simulink model "sim_discrete"  (R2018a)
settings: Solver=FixedStepAuto  StartTime=0.0  StopTime=1  FixedStep=Ti  RelTol=1e-3
undefined symbols (not defined in the file): Ad, Bd, circuit, class, Co, current_correction_start, DFd, disturbance_Ro_enable, disturbance_Ro_time, disturbance_Vin_enable, disturbance_Vin_time, h, L, Ld, NFd, opt_constant_reference, opt_dead_time, opt_equilibrium_controller, opt_pwm, opt_pwm_current_controller, opt_theorem, opt_update_equilibrium, P, pwm_limit_lower, pwm_limit_upper, pwm_period, pwm_pid_kd, pwm_pid_ki, pwm_pid_kp, pwm_pid_vc_ci, pwm_pid_vc_cp, pwm_pid_vc_vi, pwm_pid_vc_vp, pwm_sample_time, Q, R, Rc, reference_controller_initial, reference_pid_ki, reference_pid_kp, Ro, Ro_p, sensor_sample, sys, Ti, Ts, Vref, Vs, Vs_p, xe
libraries: powerlib x19, simulink x19, pePwmGenerator x2
settings Model: SimulationMode=accelerator  Creator=TARCIO-FEM  LastModifiedBy=Julio-LEPO
settings OptimizationCC: EfficientMapNaN2IntZero=off
settings HardwareCC: TargetBitPerPointer=64  TargetBitPerSizeT=64  TargetBitPerPtrDiffT=64  TargetLongLongMode=on  TargetIntDivRoundTo=Zero  TargetEndianess=LittleEndian  TargetWordSize=64  TargetHWDeviceType=MATLAB Host  ProdEqTarget=off
settings CodeAppCC: MaxIdLength=128
settings GRTTargetCC: TargetLangStandard=C89/C90 (ANSI)  CombineOutputUpdateFcns=off  GRTInterface=on

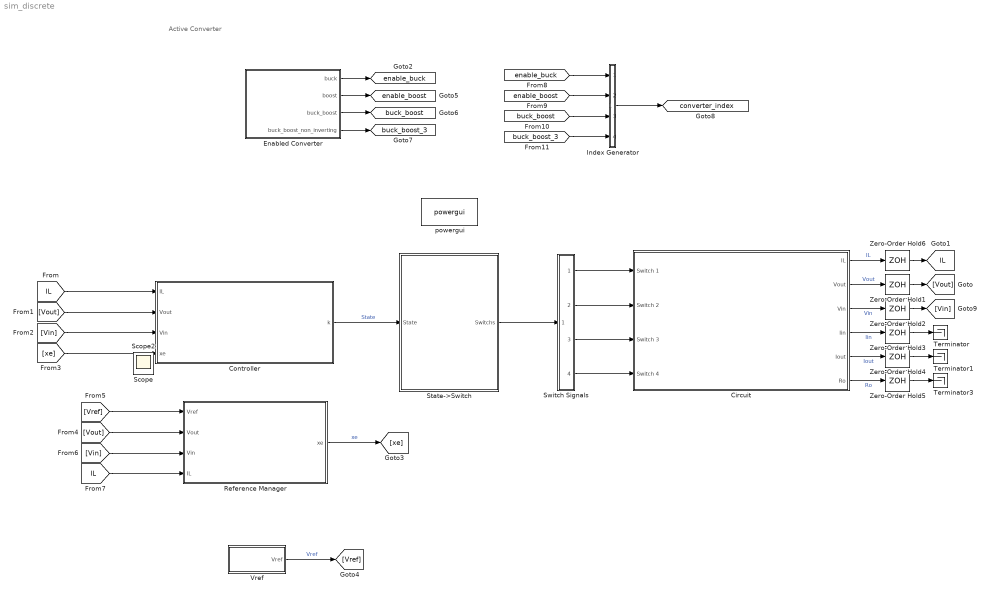
== system sim_discrete ==
  note: Active Converter
  Circuit : Subsystem
  Controller : Subsystem
  Enabled Converter : Subsystem
  Index Generator : Subsystem
  Reference Manager : Subsystem
  State->Switch : Subsystem
  Switch Signals : Subsystem
  Terminator : Terminator
  Terminator1 : Terminator
  Terminator3 : Terminator
  Vref : Subsystem
  Zero-Order Hold{1..6} (6 alike) : ZeroOrderHold  SampleTime=sensor_sample
  powergui : powerlib/powergui  Priority=1  SimulationMode=Discrete  SampleTime=Ti  frequency=60  Iterations=50  frequencyindice=0  Pbase=100e6  ErrMax=1e-4  UnitsV=kV  UnitsW=MW  buscounter=0  FunctionMessages=off  echomessages=off  EnableUseOfTLC=off  CurrentSourceSwitches=off  DisableSnubberDevices=off  DisableRonSwitches=off  DisableVfSwitches=off  DisplayEquations=off  SolverType=Tustin/Backward Euler (TBE)  Interpol=off  ExternalGateDelay=off  methode=off  Ts=100  x0status=blocks  SPID=off  SwTol=0  HookPort=off  RestoreLinks=warning  ResistiveCurrentMeasurement=off  Frange=[0:2:500]  Ylog=off  Xlog=on  ShowGrid=off  save=off  variable=ZData  structure=0  ZoomFFT=off  StartTime=0.0  cycles=1  DisplayStyle=1  fundamental=60  FreqAxis=off  MaxFrequency=1000  frequencyindicesteady=1  RmsSteady=1  display=off
  Scope : Scope
  Scope2 : Scope
  tag scope: IL=global, buck_boost=global, buck_boost_3=global, converter_index=global, enable_boost=global, enable_buck=global
  wires:
  Controller/1(k) -> State->Switch/1(State)  "State"
  [IL] -> Controller/1(IL)
  [xe] -> Controller/4(xe)
  [Vin] -> Controller/3(Vin)
  [Vout] -> Controller/2(Vout)
  Reference Manager/1(xe) -> [xe]  "xe"
  Index Generator/1(Out1) -> [converter_index]
  [Vout] -> Reference Manager/2(Vout)
  Circuit/5(Iout) -> Zero-Order Hold4/1  "Iout"
  Zero-Order Hold2/1 -> [Vin]
  Enabled Converter/3(buck_boost) -> [buck_boost]
  Switch Signals/3(S3) -> Circuit/3(Switch 3)
  [buck_boost_3] -> Index Generator/4(In4)
  Circuit/3(Vin) -> Zero-Order Hold2/1  "Vin"
  Circuit/1(IL) -> Zero-Order Hold6/1  "IL"
  Switch Signals/2(S2) -> Circuit/2(Switch 2)
  Circuit/6(Ro) -> Zero-Order Hold5/1  "Ro"
  Enabled Converter/2(boost) -> [enable_boost]
  [IL] -> Reference Manager/4(IL)
  [enable_buck] -> Index Generator/1(In1)
  [Vref] -> Reference Manager/1(Vref)
  Circuit/2(Vout) -> Zero-Order Hold1/1  "Vout"
  State->Switch/1(Switchs) -> Switch Signals/1(In1)
  Zero-Order Hold5/1 -> Terminator3/1
  Zero-Order Hold3/1 -> Terminator/1
  Switch Signals/4(S4) -> Circuit/4(Switch 4)
  Zero-Order Hold1/1 -> [Vout]
  Switch Signals/1(S1) -> Circuit/1(Switch 1)
  Vref/1(Vref) -> [Vref]  "Vref"
  Zero-Order Hold6/1 -> [IL]
  Circuit/4(Iin) -> Zero-Order Hold3/1  "Iin"
  Zero-Order Hold4/1 -> Terminator1/1
  Enabled Converter/4(buck_boost_non_inverting) -> [buck_boost_3]
  Enabled Converter/1(buck) -> [enable_buck]
  [Vin] -> Reference Manager/3(Vin)
  [enable_boost] -> Index Generator/2(In2)
  [buck_boost] -> Index Generator/3(In3)

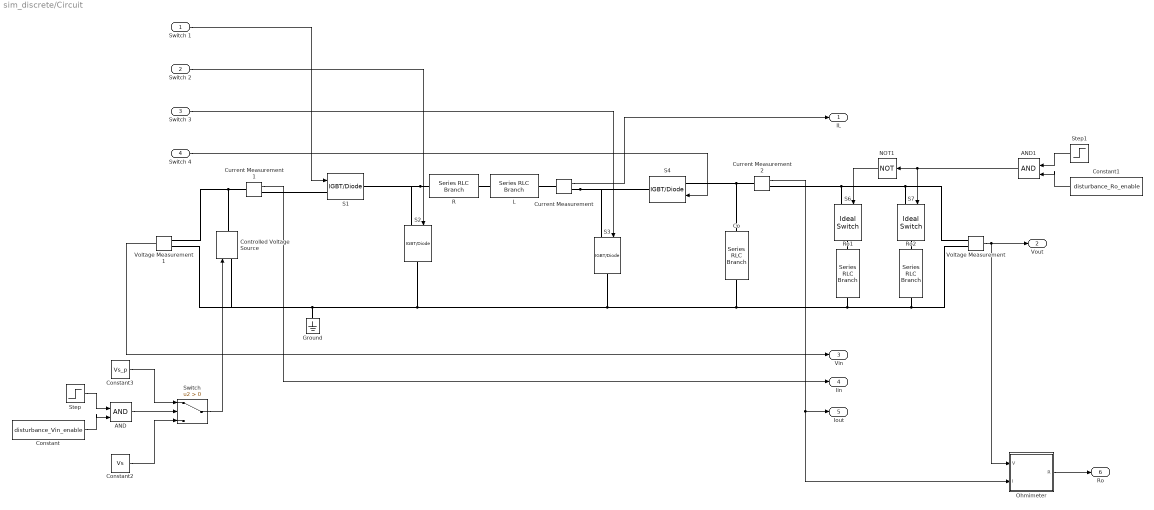
== system sim_discrete/Circuit ==
  Switch 1 : Inport
  Switch 2 : Inport  Port=2
  Switch 3 : Inport  Port=3
  Switch 4 : Inport  Port=4
  AND : Logic  IconShape=distinctive  AllPortsSameDT=off  OutDataTypeStr=boolean
  AND1 : Logic  IconShape=distinctive  AllPortsSameDT=off  OutDataTypeStr=boolean
  Co : powerlib/Elements/Series RLC Branch  LConnTagsString=__new0  RConnTagsString=__new0  BranchType=RC  Resistance=Rc  Inductance=L  SetiL0=off  InitialCurrent=0  Capacitance=Co  Setx0=off  InitialVoltage=0  Measurements=None
  Constant : Constant  Value=disturbance_Vin_enable
  Constant1 : Constant  Value=disturbance_Ro_enable
  Constant2 : Constant  Value=Vs
  Constant3 : Constant  Value=Vs_p
  Controlled Voltage Source : powerlib/Electrical Sources/Controlled Voltage Source  Initialize=on  Source_Type=DC  Amplitude=0  Phase=0  Frequency=0  Measurements=None
  Current Measurement : powerlib/Measurements/Current Measurement  PhasorSimulation=off  OutputType=Complex  PSBequivalent=0
  Current Measurement1 : powerlib/Measurements/Current Measurement  PhasorSimulation=off  OutputType=Complex  PSBequivalent=0
  Current Measurement2 : powerlib/Measurements/Current Measurement  PhasorSimulation=off  OutputType=Complex  PSBequivalent=0
  Ground : powerlib/Elements/Ground  LConnTagsString=a
  L : powerlib/Elements/Series RLC Branch  LConnTagsString=__new0  RConnTagsString=__new0  BranchType=L  Resistance=1  Inductance=L  SetiL0=off  InitialCurrent=0  Capacitance=1e-6  Setx0=off  InitialVoltage=0  Measurements=None
  NOT1 : Logic  Operator=NOT  IconShape=distinctive  AllPortsSameDT=off  OutDataTypeStr=boolean
  Ohmimeter : Subsystem
  R : powerlib/Elements/Series RLC Branch  LConnTagsString=__new0  RConnTagsString=__new0  BranchType=R  Resistance=R  Inductance=1e-3  SetiL0=off  InitialCurrent=0  Capacitance=1e-6  Setx0=off  InitialVoltage=0  Measurements=None
  Ro1 : powerlib/Elements/Series RLC Branch  LConnTagsString=__new0  RConnTagsString=__new0  BranchType=R  Resistance=Ro  Inductance=1e-3  SetiL0=off  InitialCurrent=0  Capacitance=1e-6  Setx0=off  InitialVoltage=0  Measurements=None
  Ro2 : powerlib/Elements/Series RLC Branch  LConnTagsString=__new0  RConnTagsString=__new0  BranchType=R  Resistance=Ro_p  Inductance=1e-3  SetiL0=off  InitialCurrent=0  Capacitance=1e-6  Setx0=off  InitialVoltage=0  Measurements=None
  S{1..4} (4 alike) : powerlib/Power Electronics/IGBT//Diode  Ron=1e-3  Rs=1e5  Cs=inf  Measurements=off
  S6 : powerlib/Power Electronics/Ideal Switch  Ron=0.001  Lon=0  IC=0  Rs=1e5  Cs=inf  Measurements=off
  S7 : powerlib/Power Electronics/Ideal Switch  Ron=0.001  Lon=0  IC=0  Rs=1e5  Cs=inf  Measurements=off
  Step : Step  Time=disturbance_Vin_time  SampleTime=0
  Step1 : Step  Time=disturbance_Ro_time  SampleTime=0
  Switch : Switch  Criteria=u2 > Threshold
  Voltage Measurement : powerlib/Measurements/Voltage Measurement  PhasorSimulation=off  OutputType=Complex  PSBequivalent=0
  Voltage Measurement1 : powerlib/Measurements/Voltage Measurement  PhasorSimulation=off  OutputType=Complex  PSBequivalent=0
  IL : Outport
  Vout : Outport  Port=2
  Vin : Outport  Port=3
  Iin : Outport  Port=4
  Iout : Outport  Port=5
  Ro : Outport  Port=6
  wires:
  Switch 1/1 -> S1/1
  Voltage Measurement1/1 -> Vin/1
  Switch 2/1 -> S2/1
  Constant1/1 -> AND1/2
  AND1/1 -> S7/1, NOT1/1
  NOT1/1 -> S6/1
  Step1/1 -> AND1/1
  AND/1 -> Switch/2
  Constant/1 -> AND/2
  Step/1 -> AND/1
  Constant2/1 -> Switch/3
  Constant3/1 -> Switch/1
  Current Measurement1/1 -> Iin/1
  Current Measurement/1 -> IL/1
  Switch/1 -> Controlled Voltage Source/1
  Switch 4/1 -> S4/1
  Switch 3/1 -> S3/1
  Voltage Measurement/1 -> Vout/1, Ohmimeter/1(V)
  Ohmimeter/1(R) -> Ro/1
  Current Measurement2/1 -> Ohmimeter/2(I), Iout/1
  connections:
  L/LConn1 -- R/RConn1
  R/LConn1 -- S2/LConn1 -- S1/RConn1
  Current Measurement/LConn1 -- L/RConn1
  Current Measurement2/LConn1 -- S4/LConn1 -- Co/LConn1
  Voltage Measurement/LConn2 -- Ro2/RConn1 -- Ro1/RConn1 -- S3/RConn1 -- S2/RConn1 -- Voltage Measurement1/LConn2 -- Controlled Voltage Source/LConn1 -- Ground/LConn1 -- Co/RConn1
  S7/RConn1 -- Ro2/LConn1
  S6/RConn1 -- Ro1/LConn1
  Current Measurement1/LConn1 -- Controlled Voltage Source/RConn1 -- Voltage Measurement1/LConn1
  S1/LConn1 -- Current Measurement1/RConn1
  S6/LConn1 -- Current Measurement2/RConn1 -- S7/LConn1 -- Voltage Measurement/LConn1
  Current Measurement/RConn1 -- S4/RConn1 -- S3/LConn1

== system sim_discrete/Controller ==
  IL : Inport
  Vout : Inport  Port=2
  Vin : Inport  Port=3
  xe : Inport  Port=4
  Constant : Constant  Value=opt_pwm
  Discrete Switched Control : Subsystem
  PWM Control : Subsystem
  Selector : Selector  InputPortWidth=2  IndexOptions=Index vector (dialog)  Indices=[2]  OutputSizes=1
  Switch : Switch  Criteria=u2 > Threshold
  k : Outport
  wires:
  IL/1 -> PWM Control/3(IL), Discrete Switched Control/1(IL)
  Vout/1 -> PWM Control/2(Vout), Discrete Switched Control/2(Vout)
  Vin/1 -> Discrete Switched Control/3(Vin)
  Switch/1 -> k/1
  Discrete Switched Control/1(k) -> Switch/3  "Switched Control K"
  Constant/1 -> Switch/2
  xe/1 -> Discrete Switched Control/4(xe), Selector/1
  Selector/1 -> PWM Control/1(Vref)
  PWM Control/1(k) -> Switch/1  "PWM K"

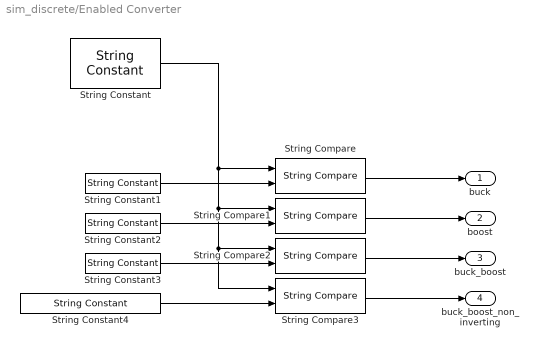
== system sim_discrete/Enabled Converter ==
  String Compare{,1..3} (4 alike) : StringCompare
  String Constant : StringConstant  String=class(circuit)
  String Constant1 : StringConstant  String='buck'
  String Constant2 : StringConstant  String='boost'
  String Constant3 : StringConstant  String='buck_boost'
  String Constant4 : StringConstant  String='buck_boost_non_inverting'
  buck : Outport
  boost : Outport  Port=2
  buck_boost : Outport  Port=3
  buck_boost_non_inverting : Outport  Port=4
  wires:
  String Constant1/1 -> String Compare/2
  String Constant/1 -> String Compare/1, String Compare1/1, String Compare2/1, String Compare3/1
  String Constant3/1 -> String Compare2/2
  String Compare2/1 -> buck_boost/1
  String Compare1/1 -> boost/1
  String Constant4/1 -> String Compare3/2
  String Compare3/1 -> buck_boost_non_inverting/1
  String Compare/1 -> buck/1
  String Constant2/1 -> String Compare1/2

== system sim_discrete/Index Generator ==
  In1 : Inport
  In2 : Inport  Port=2
  In3 : Inport  Port=3
  In4 : Inport  Port=4
  Gain : Gain
  Gain1 : Gain  Gain=2
  Gain2 : Gain  Gain=3
  Gain3 : Gain  Gain=4
  Sum : Sum  Inputs=++++
  Out1 : Outport
  wires:
  Gain/1 -> Sum/1
  In3/1 -> Gain2/1
  In2/1 -> Gain1/1
  Gain1/1 -> Sum/2
  Sum/1 -> Out1/1
  Gain2/1 -> Sum/3
  In4/1 -> Gain3/1
  Gain3/1 -> Sum/4
  In1/1 -> Gain/1

== system sim_discrete/Reference Manager ==
  Vref : Inport
  Vout : Inport  Port=2
  Vin : Inport  Port=3
  IL : Inport  Port=4
  Constant : Constant  Value=xe
  Reference Update : Subsystem
  Switch : Switch  Criteria=u2 > Threshold
  opt_update_equilibrium : Constant  Value=opt_update_equilibrium
  xe : Outport
  wires:
  Vout/1 -> Reference Update/2(Vout)
  Vin/1 -> Reference Update/3(Vin)
  Vref/1 -> Reference Update/1(Vref)
  opt_update_equilibrium/1 -> Switch/2
  Switch/1 -> xe/1
  Reference Update/1(xe) -> Switch/1  "xe"
  Constant/1 -> Switch/3
  IL/1 -> Reference Update/4(IL)

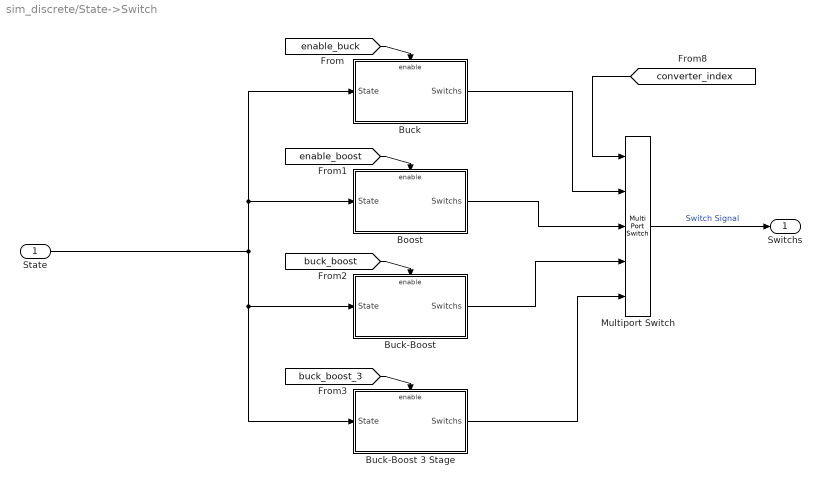
== system sim_discrete/State->Switch ==
  State : Inport
  Boost : Subsystem
  Buck : Subsystem
  Buck-Boost : Subsystem
  Buck-Boost 3 Stage : Subsystem
  Multiport Switch : MultiPortSwitch  Inputs=4
  Switchs : Outport
  wires:
  State/1 -> Buck-Boost/1(State), Buck-Boost 3 Stage/1(State), Boost/1(State), Buck/1(State)
  Buck/1(Switchs) -> Multiport Switch/2
  Boost/1(Switchs) -> Multiport Switch/3
  Buck-Boost 3 Stage/1(Switchs) -> Multiport Switch/5
  Buck-Boost/1(Switchs) -> Multiport Switch/4
  [enable_buck] -> Buck/Enable
  [enable_boost] -> Boost/Enable
  [buck_boost] -> Buck-Boost/Enable
  [buck_boost_3] -> Buck-Boost 3 Stage/Enable
  Multiport Switch/1 -> Switchs/1  "Switch Signal"
  [converter_index] -> Multiport Switch/1

== system sim_discrete/Switch Signals ==
  In1 : Inport
  Constant : Constant  Value=opt_dead_time
  Dead Time : Subsystem
  Demux : Demux
  Scope : Scope  NumInputPorts=2
  Switch : Switch  Criteria=u2 > Threshold
  S1 : Outport
  S2 : Outport  Port=2
  S3 : Outport  Port=3
  S4 : Outport  Port=4
  wires:
  Constant/1 -> Dead Time/Enable, Switch/2
  Dead Time/1(Out1) -> Scope/2, Switch/1
  In1/1 -> Scope/1, Dead Time/1(In1), Switch/3
  Demux/2 -> S2/1
  Demux/1 -> S1/1
  Demux/4 -> S4/1
  Demux/3 -> S3/1
  Switch/1 -> Demux/1

== system sim_discrete/Vref ==
  Constant Reference : Subsystem
  Switch1 : Switch  Criteria=u2 > Threshold
  Variable Reference : Subsystem
  opt_constant_reference : Constant  Value=opt_constant_reference
  Vref : Outport
  wires:
  opt_constant_reference/1 -> Switch1/2
  Switch1/1 -> Vref/1
  Variable Reference/1(Vref) -> Switch1/3
  Constant Reference/1(Vref) -> Switch1/1

== system sim_discrete/Circuit/Ohmimeter ==
  V : Inport
  I : Inport  Port=2
  Compare To Zero : simulink/Logic and Bit Operations/Compare To Zero  relop=~=  OutDataTypeStr=boolean
  Constant4 : Constant  Value=Ro
  Divide : Product  Inputs=*/
  One : Constant
  Switch1 : Switch  Criteria=u2 ~= 0
  Switch2 : Switch  Criteria=u2 ~= 0
  R : Outport
  wires:
  Compare To Zero/1 -> Switch1/2, Switch2/2
  I/1 -> Switch1/1, Compare To Zero/1
  Divide/1 -> Switch2/1
  Constant4/1 -> Switch2/3
  Switch1/1 -> Divide/2
  One/1 -> Switch1/3
  V/1 -> Divide/1
  Switch2/1 -> R/1

== system sim_discrete/Controller/Discrete Switched Control ==
  IL : Inport
  Vout : Inport  Port=2
  Vin : Inport  Port=3
  xe : Inport  Port=4
  Discrete Switching Strategy : MATLAB Function  TreatAsAtomicUnit=on
  Mux : Mux  Inputs=2
  System Properties : Subsystem
  Zero-Order Hold : ZeroOrderHold  SampleTime=Ts
  k : Outport
  wires:
  Vin/1 -> Discrete Switching Strategy/4(u)
  Discrete Switching Strategy/1(k) -> Zero-Order Hold/1
  System Properties/1(theorem) -> Discrete Switching Strategy/1(theorem)
  System Properties/2(sys) -> Discrete Switching Strategy/2(sys)
  Mux/1 -> Discrete Switching Strategy/3(x)
  IL/1 -> Mux/1
  Vout/1 -> Mux/2
  xe/1 -> Discrete Switching Strategy/5(xe)
  Zero-Order Hold/1 -> k/1

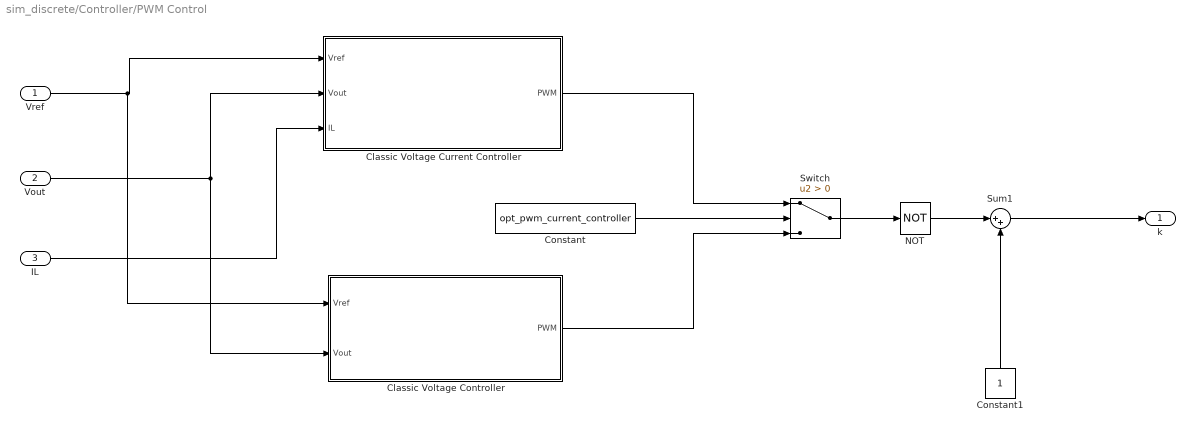
== system sim_discrete/Controller/PWM Control ==
  Vref : Inport
  Vout : Inport  Port=2
  IL : Inport  Port=3
  Classic Voltage Controller : Subsystem
  Classic Voltage Current Controller : Subsystem
  Constant : Constant  Value=opt_pwm_current_controller
  Constant1 : Constant
  NOT : Logic  Operator=NOT  IconShape=distinctive  AllPortsSameDT=off  OutDataTypeStr=boolean
  Sum1 : Sum  Inputs=|++
  Switch : Switch  Criteria=u2 > Threshold
  k : Outport
  wires:
  Sum1/1 -> k/1
  NOT/1 -> Sum1/1
  Constant1/1 -> Sum1/2
  Vref/1 -> Classic Voltage Controller/1(Vref), Classic Voltage Current Controller/1(Vref)
  Vout/1 -> Classic Voltage Controller/2(Vout), Classic Voltage Current Controller/2(Vout)
  IL/1 -> Classic Voltage Current Controller/3(IL)
  Constant/1 -> Switch/2
  Switch/1 -> NOT/1
  Classic Voltage Controller/1(PWM) -> Switch/3
  Classic Voltage Current Controller/1(PWM) -> Switch/1

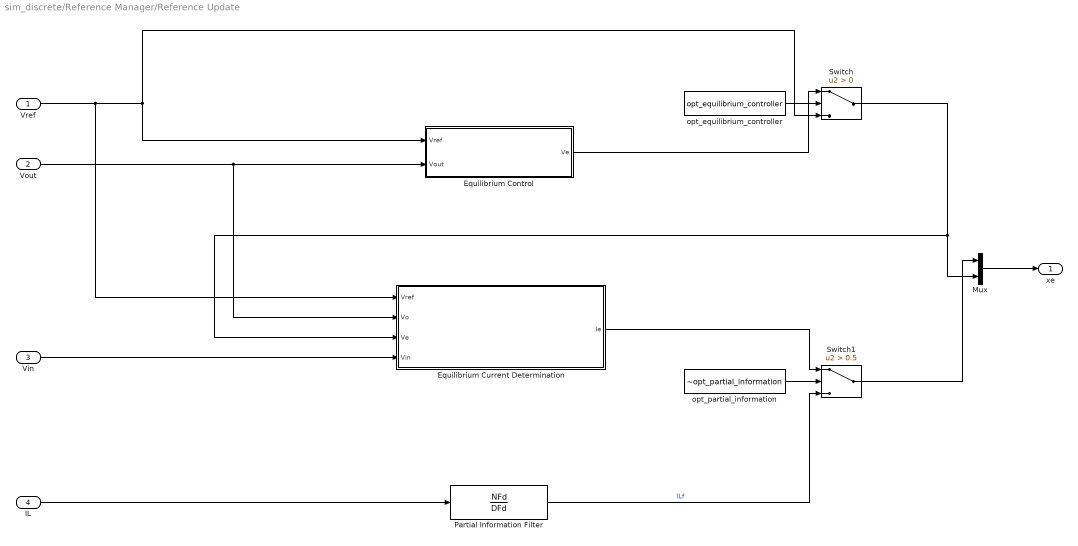
== system sim_discrete/Reference Manager/Reference Update ==
  Vref : Inport
  Vout : Inport  Port=2
  Vin : Inport  Port=3
  IL : Inport  Port=4
  Equilibrium Control : Subsystem
  Equilibrium Current Determination : Subsystem
  Mux : Mux  Inputs=2
  Partial Information Filter : DiscreteTransferFcn  Numerator=NFd  Denominator=DFd  SampleTime=1e-3
  Switch : Switch  Criteria=u2 > Threshold
  Switch1 : Switch  Criteria=u2 > Threshold  Threshold=0.5
  opt_equilibrium_controller : Constant  Value=opt_equilibrium_controller
  opt_partial_information : Constant  Value=~opt_partial_information
  xe : Outport
  wires:
  Vref/1 -> Equilibrium Current Determination/1(Vref), Equilibrium Control/1(Vref), Switch/3
  Mux/1 -> xe/1
  opt_equilibrium_controller/1 -> Switch/2
  Switch/1 -> Equilibrium Current Determination/3(Ve), Mux/2
  Switch1/1 -> Mux/1
  opt_partial_information/1 -> Switch1/2
  Partial Information Filter/1 -> Switch1/3  "ILf"
  IL/1 -> Partial Information Filter/1
  Vout/1 -> Equilibrium Current Determination/2(Vo), Equilibrium Control/2(Vout)
  Equilibrium Control/1(Ve) -> Switch/1
  Vin/1 -> Equilibrium Current Determination/4(Vin)
  Equilibrium Current Determination/1(Ie) -> Switch1/1

== system sim_discrete/State->Switch/Boost ==
  State : Inport
  Enable : EnablePort
  Compare To Constant : simulink/Logic and Bit Operations/Compare To Constant  relop=<=  const=1.5  OutDataTypeStr=boolean
  Constant : Constant  Value=false
  Constant1 : Constant  Value=true
  Mux : Mux
  NOT : Logic  Operator=NOT  IconShape=distinctive  AllPortsSameDT=off  OutDataTypeStr=boolean
  Switchs : Outport
  wires:
  Mux/1 -> Switchs/1
  Compare To Constant/1 -> Mux/3, NOT/1
  State/1 -> Compare To Constant/1
  NOT/1 -> Mux/4
  Constant1/1 -> Mux/1
  Constant/1 -> Mux/2

== system sim_discrete/State->Switch/Buck ==
  State : Inport
  Enable : EnablePort
  Compare To Constant : simulink/Logic and Bit Operations/Compare To Constant  relop=<=  const=1.5  OutDataTypeStr=boolean
  Constant : Constant  Value=false
  Constant1 : Constant  Value=true
  Mux : Mux
  NOT : Logic  Operator=NOT  IconShape=distinctive  AllPortsSameDT=off  OutDataTypeStr=boolean
  Switchs : Outport
  wires:
  Mux/1 -> Switchs/1
  Compare To Constant/1 -> Mux/1, NOT/1
  Constant1/1 -> Mux/4
  NOT/1 -> Mux/2
  Constant/1 -> Mux/3
  State/1 -> Compare To Constant/1

== system sim_discrete/State->Switch/Buck-Boost ==
  State : Inport
  Enable : EnablePort
  Compare To Constant : simulink/Logic and Bit Operations/Compare To Constant  relop=<=  const=1.5  OutDataTypeStr=boolean
  Mux : Mux
  NOT : Logic  Operator=NOT  IconShape=distinctive  AllPortsSameDT=off  OutDataTypeStr=boolean
  Switchs : Outport
  wires:
  Mux/1 -> Switchs/1
  Compare To Constant/1 -> Mux/3, Mux/1, NOT/1
  NOT/1 -> Mux/4, Mux/2
  State/1 -> Compare To Constant/1

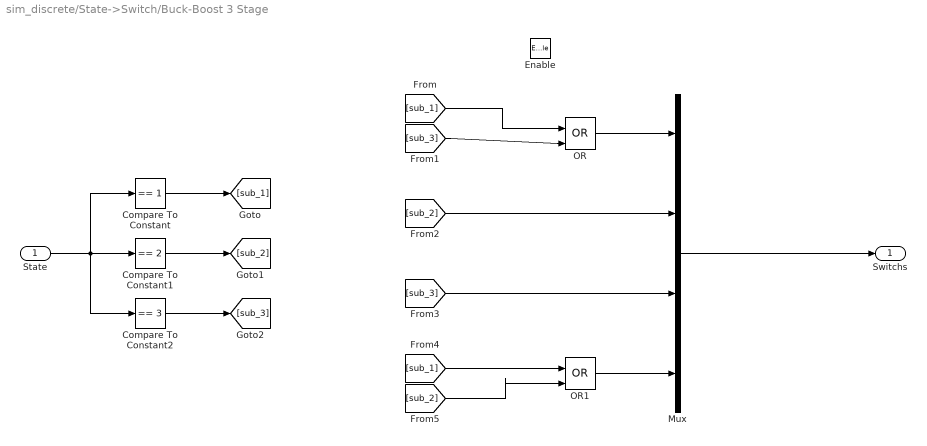
== system sim_discrete/State->Switch/Buck-Boost 3 Stage ==
  State : Inport
  Enable : EnablePort
  Compare To Constant : simulink/Logic and Bit Operations/Compare To Constant  relop===  const=1  OutDataTypeStr=boolean
  Compare To Constant1 : simulink/Logic and Bit Operations/Compare To Constant  relop===  const=2  OutDataTypeStr=boolean
  Compare To Constant2 : simulink/Logic and Bit Operations/Compare To Constant  relop===  const=3  OutDataTypeStr=boolean
  Mux : Mux
  OR : Logic  Operator=OR  IconShape=distinctive  AllPortsSameDT=off  OutDataTypeStr=boolean
  OR1 : Logic  Operator=OR  IconShape=distinctive  AllPortsSameDT=off  OutDataTypeStr=boolean
  Switchs : Outport
  wires:
  Mux/1 -> Switchs/1
  [sub_1] -> OR/1
  [sub_1] -> OR1/1
  [sub_2] -> Mux/2
  [sub_2] -> OR1/2
  State/1 -> Compare To Constant2/1, Compare To Constant1/1, Compare To Constant/1
  OR1/1 -> Mux/4
  [sub_3] -> OR/2
  [sub_3] -> Mux/3
  Compare To Constant/1 -> [sub_1]
  Compare To Constant2/1 -> [sub_3]
  OR/1 -> Mux/1
  Compare To Constant1/1 -> [sub_2]

== system sim_discrete/Switch Signals/Dead Time ==
  In1 : Inport
  Enable : EnablePort
  Dead Time : Subsystem
  Dead Time1 : Subsystem
  Dead Time2 : Subsystem
  Dead Time3 : Subsystem
  Demux : Demux
  Mux : Mux
  Out1 : Outport
  wires:
  Demux/4 -> Dead Time3/1(Signal)
  Demux/3 -> Dead Time2/1(Signal)
  Demux/2 -> Dead Time1/1(Signal)
  Demux/1 -> Dead Time/1(Signal)
  In1/1 -> Demux/1
  Dead Time3/1(Signal Delayed) -> Mux/4
  Dead Time2/1(Signal Delayed) -> Mux/3
  Dead Time1/1(Signal Delayed) -> Mux/2
  Dead Time/1(Signal Delayed) -> Mux/1
  Mux/1 -> Out1/1

== system sim_discrete/Vref/Constant Reference ==
  Constant : Constant  Value=Vref
  Vref : Outport
  wires:
  Constant/1 -> Vref/1

== system sim_discrete/Vref/Variable Reference ==
  Constant : Constant  Value=Vref
  Rate Limiter : RateLimiter  RisingSlewLimit=10  FallingSlewLimit=-10  SampleTimeMode=inherited
  Step : Step  Time=1.5  After=20  SampleTime=0
  Sum : Sum  Inputs=|++
  Vref : Outport
  wires:
  Constant/1 -> Sum/1
  Sum/1 -> Vref/1
  Step/1 -> Rate Limiter/1
  Rate Limiter/1 -> Sum/2

== system sim_discrete/Controller/Discrete Switched Control/System Properties ==
  Bus Creator : BusCreator  Inputs=7  OutDataTypeStr=Bus: SystemDataBus
  Constant : Constant  Value=Ad  VectorParams1D=off
  Constant1 : Constant  Value=Bd  VectorParams1D=off
  Constant2 : Constant  Value=P  VectorParams1D=off
  Constant3 : Constant  Value=Q  VectorParams1D=off
  Constant4 : Constant  Value=h  VectorParams1D=off
  Constant5 : Constant  Value=sys.N
  Constant6 : Constant  Value=opt_theorem
  Constant7 : Constant  Value=Ld  VectorParams1D=off
  theorem : Outport
  sys : Outport  Port=2
  wires:
  Bus Creator/1 -> sys/1
  Constant2/1 -> Bus Creator/3  "P"
  Constant1/1 -> Bus Creator/2  "B"
  Constant/1 -> Bus Creator/1  "A"
  Constant3/1 -> Bus Creator/4  "Q"
  Constant5/1 -> Bus Creator/5  "N"
  Constant6/1 -> theorem/1
  Constant4/1 -> Bus Creator/6  "h"
  Constant7/1 -> Bus Creator/7  "L"

== system sim_discrete/Controller/PWM Control/Classic Voltage Controller ==
  Vref : Inport
  Vout : Inport  Port=2
  PID Controller : simulink/Continuous/PID Controller  Controller=PI  TimeDomain=Discrete-time  SampleTime=pwm_period  IntegratorMethod=Forward Euler  FilterMethod=Forward Euler  Form=Parallel  UseFilter=on  ControllerParametersSource=internal  P=pwm_pid_kp  I=pwm_pid_ki  D=pwm_pid_kd  N=100  InitialConditionSource=internal  InitialConditionForIntegrator=0  InitialConditionForFilter=0  ExternalReset=none  LimitOutput=off  UpperSaturationLimit=inf  LowerSaturationLimit=-inf  LinearizeAsGain=on  AntiWindupMode=none  Kb=1  TrackingMode=off  Kt=1  PParamMin=[]  PParamMax=[]  IParamMin=[]  IParamMax=[]  DParamMin=[]  DParamMax=[]  NParamMin=[]  NParamMax=[]  KbParamMin=[]  KbParamMax=[]  KtParamMin=[]  KtParamMax=[]  POutMin=[]  POutMax=[]  IOutMin=[]  IOutMax=[]  DOutMin=[]  DOutMax=[]  NOutMin=[]  NOutMax=[]  KbOutMin=[]  KbOutMax=[]  KtOutMin=[]  KtOutMax=[]  IntegratorOutMin=[]  IntegratorOutMax=[]  FilterOutMin=[]  FilterOutMax=[]  SumOutMin=[]  SumOutMax=[]  SumI1OutMin=[]  SumI1OutMax=[]  SumI2OutMin=[]  SumI2OutMax=[]  SumI3OutMin=[]  SumI3OutMax=[]  SumDOutMin=[]  SumDOutMax=[]  SaturationOutMin=[]  SaturationOutMax=[]  IntegratorContinuousStateAttributes=''  IntegratorStateMustResolveToSignalObject=off  IntegratorRTWStateStorageClass=Auto  FilterContinuousStateAttributes=''  FilterStateMustResolveToSignalObject=off  FilterRTWStateStorageClass=Auto  DifferentiatorICPrevScaledInput=0  DifferentiatorOutMin=[]  DifferentiatorOutMax=[]  FilterDiffOutCoefMin=[]  FilterDiffOutCoefMax=[]  SumDenOutMin=[]  SumDenOutMax=[]  SumNumOutMin=[]  SumNumOutMax=[]  ReciprocalOutMin=[]  ReciprocalOutMax=[]  DivideOutMin=[]  DivideOutMax=[]  TunerSelectOption=Transfer Function Based (PID Tuner App)
  PWM Generator : pePwmGenerator/PWM Generator  CarrCount=Up  Tper=pwm_period  Ts=pwm_sample_time
  Saturation : Saturate  UpperLimit=pwm_limit_upper  LowerLimit=pwm_limit_lower
  Sum : Sum  Inputs=|+-
  PWM : Outport
  wires:
  Saturation/1 -> PWM Generator/1  "PWM Duty Cycle"
  PWM Generator/1 -> PWM/1
  PID Controller/1 -> Saturation/1
  Sum/1 -> PID Controller/1
  Vref/1 -> Sum/1
  Vout/1 -> Sum/2

== system sim_discrete/Controller/PWM Control/Classic Voltage Current Controller ==
  Vref : Inport
  Vout : Inport  Port=2
  IL : Inport  Port=3
  Current Controller : simulink/Continuous/PID Controller  Controller=PI  TimeDomain=Discrete-time  SampleTime=pwm_period  IntegratorMethod=Forward Euler  FilterMethod=Forward Euler  Form=Parallel  UseFilter=on  ControllerParametersSource=internal  P=pwm_pid_vc_cp  I=pwm_pid_vc_ci  D=pwm_pid_kd  N=100  InitialConditionSource=internal  InitialConditionForIntegrator=0  InitialConditionForFilter=0  ExternalReset=none  LimitOutput=off  UpperSaturationLimit=inf  LowerSaturationLimit=-inf  LinearizeAsGain=on  AntiWindupMode=none  Kb=1  TrackingMode=off  Kt=1  PParamMin=[]  PParamMax=[]  IParamMin=[]  IParamMax=[]  DParamMin=[]  DParamMax=[]  NParamMin=[]  NParamMax=[]  KbParamMin=[]  KbParamMax=[]  KtParamMin=[]  KtParamMax=[]  POutMin=[]  POutMax=[]  IOutMin=[]  IOutMax=[]  DOutMin=[]  DOutMax=[]  NOutMin=[]  NOutMax=[]  KbOutMin=[]  KbOutMax=[]  KtOutMin=[]  KtOutMax=[]  IntegratorOutMin=[]  IntegratorOutMax=[]  FilterOutMin=[]  FilterOutMax=[]  SumOutMin=[]  SumOutMax=[]  SumI1OutMin=[]  SumI1OutMax=[]  SumI2OutMin=[]  SumI2OutMax=[]  SumI3OutMin=[]  SumI3OutMax=[]  SumDOutMin=[]  SumDOutMax=[]  SaturationOutMin=[]  SaturationOutMax=[]  IntegratorContinuousStateAttributes=''  IntegratorStateMustResolveToSignalObject=off  IntegratorRTWStateStorageClass=Auto  FilterContinuousStateAttributes=''  FilterStateMustResolveToSignalObject=off  FilterRTWStateStorageClass=Auto  DifferentiatorICPrevScaledInput=0  DifferentiatorOutMin=[]  DifferentiatorOutMax=[]  FilterDiffOutCoefMin=[]  FilterDiffOutCoefMax=[]  SumDenOutMin=[]  SumDenOutMax=[]  SumNumOutMin=[]  SumNumOutMax=[]  ReciprocalOutMin=[]  ReciprocalOutMax=[]  DivideOutMin=[]  DivideOutMax=[]  TunerSelectOption=Transfer Function Based (PID Tuner App)
  PWM Generator : pePwmGenerator/PWM Generator  CarrCount=Up  Tper=pwm_period  Ts=pwm_sample_time
  Saturation : Saturate  UpperLimit=pwm_limit_upper  LowerLimit=pwm_limit_lower
  Sum : Sum  Inputs=|+-
  Sum2 : Sum  Inputs=|+-
  Voltage Controller : simulink/Continuous/PID Controller  Controller=PI  TimeDomain=Discrete-time  SampleTime=pwm_period  IntegratorMethod=Forward Euler  FilterMethod=Forward Euler  Form=Parallel  UseFilter=on  ControllerParametersSource=internal  P=pwm_pid_vc_vp  I=pwm_pid_vc_vi  D=0  N=100  InitialConditionSource=internal  InitialConditionForIntegrator=0  InitialConditionForFilter=0  ExternalReset=none  LimitOutput=off  UpperSaturationLimit=inf  LowerSaturationLimit=-inf  LinearizeAsGain=on  AntiWindupMode=none  Kb=1  TrackingMode=off  Kt=1  PParamMin=[]  PParamMax=[]  IParamMin=[]  IParamMax=[]  DParamMin=[]  DParamMax=[]  NParamMin=[]  NParamMax=[]  KbParamMin=[]  KbParamMax=[]  KtParamMin=[]  KtParamMax=[]  POutMin=[]  POutMax=[]  IOutMin=[]  IOutMax=[]  DOutMin=[]  DOutMax=[]  NOutMin=[]  NOutMax=[]  KbOutMin=[]  KbOutMax=[]  KtOutMin=[]  KtOutMax=[]  IntegratorOutMin=[]  IntegratorOutMax=[]  FilterOutMin=[]  FilterOutMax=[]  SumOutMin=[]  SumOutMax=[]  SumI1OutMin=[]  SumI1OutMax=[]  SumI2OutMin=[]  SumI2OutMax=[]  SumI3OutMin=[]  SumI3OutMax=[]  SumDOutMin=[]  SumDOutMax=[]  SaturationOutMin=[]  SaturationOutMax=[]  IntegratorContinuousStateAttributes=''  IntegratorStateMustResolveToSignalObject=off  IntegratorRTWStateStorageClass=Auto  FilterContinuousStateAttributes=''  FilterStateMustResolveToSignalObject=off  FilterRTWStateStorageClass=Auto  DifferentiatorICPrevScaledInput=0  DifferentiatorOutMin=[]  DifferentiatorOutMax=[]  FilterDiffOutCoefMin=[]  FilterDiffOutCoefMax=[]  SumDenOutMin=[]  SumDenOutMax=[]  SumNumOutMin=[]  SumNumOutMax=[]  ReciprocalOutMin=[]  ReciprocalOutMax=[]  DivideOutMin=[]  DivideOutMax=[]  TunerSelectOption=Transfer Function Based (PID Tuner App)
  PWM : Outport
  wires:
  Sum2/1 -> Current Controller/1
  Sum/1 -> Voltage Controller/1
  Vout/1 -> Sum/2
  Voltage Controller/1 -> Sum2/1
  IL/1 -> Sum2/2
  Current Controller/1 -> Saturation/1
  Vref/1 -> Sum/1
  Saturation/1 -> PWM Generator/1  "PWM Duty Cycle"
  PWM Generator/1 -> PWM/1

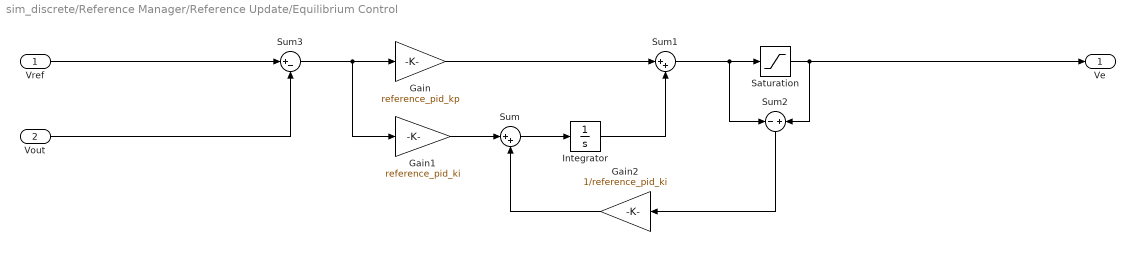
== system sim_discrete/Reference Manager/Reference Update/Equilibrium Control ==
  Vref : Inport
  Vout : Inport  Port=2
  Gain : Gain  Gain=reference_pid_kp
  Gain1 : Gain  Gain=reference_pid_ki
  Gain2 : Gain  Gain=1/reference_pid_ki
  Integrator : Integrator  InitialCondition=reference_controller_initial
  Saturation : Saturate  UpperLimit=400  LowerLimit=0
  Sum : Sum  Inputs=|++
  Sum1 : Sum  Inputs=|++
  Sum2 : Sum  Inputs=-|+
  Sum3 : Sum  Inputs=|+-
  Ve : Outport
  wires:
  Sum1/1 -> Sum2/1, Saturation/1
  Sum/1 -> Integrator/1
  Gain1/1 -> Sum/1
  Integrator/1 -> Sum1/2
  Vout/1 -> Sum3/2
  Sum3/1 -> Gain1/1, Gain/1
  Gain/1 -> Sum1/1
  Gain2/1 -> Sum/2
  Saturation/1 -> Ve/1, Sum2/2
  Sum2/1 -> Gain2/1
  Vref/1 -> Sum3/1

== system sim_discrete/Reference Manager/Reference Update/Equilibrium Current Determination ==
  Vref : Inport
  Vo : Inport  Port=2
  Ve : Inport  Port=3
  Vin : Inport  Port=4
  Current Correction : Subsystem
  Current Estimation : Subsystem
  Switch2 : Switch  Criteria=u2 > Threshold  Threshold=0.5
  opt_current_correction : Constant  Value=~opt_current_correction
  Ie : Outport
  wires:
  Ve/1 -> Current Estimation/1(Ve)
  Current Correction/1(Ie) -> Switch2/3
  Switch2/1 -> Ie/1
  opt_current_correction/1 -> Switch2/2
  Current Estimation/1(Ie) -> Current Correction/1(IL_e), Switch2/1
  Vref/1 -> Current Correction/2(Vref)
  Vin/1 -> Current Estimation/2(Vin)
  Vo/1 -> Current Correction/3(Vo)

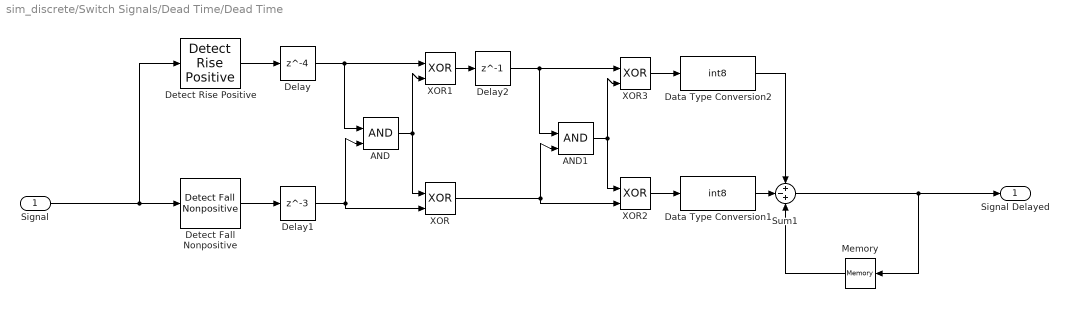
== system sim_discrete/Switch Signals/Dead Time/Dead Time ==
  Signal : Inport
  AND : Logic  IconShape=distinctive  AllPortsSameDT=off  OutDataTypeStr=boolean
  AND1 : Logic  IconShape=distinctive  AllPortsSameDT=off  OutDataTypeStr=boolean
  Data Type Conversion1 : DataTypeConversion  OutDataTypeStr=int8
  Data Type Conversion2 : DataTypeConversion  OutDataTypeStr=int8
  Delay : Delay  DelayLength=4
  Delay1 : Delay  DelayLength=3
  Delay2 : Delay  DelayLength=1
  Detect Fall Nonpositive : simulink/Logic and Bit Operations/Detect Fall Nonpositive  vinit=true  OutDataTypeStr=boolean
      settings: SourceProductName=Simulink  SourceProductBaseCode=SL
  Detect Rise Positive : simulink/Logic and Bit Operations/Detect Rise Positive  vinit=0  OutDataTypeStr=boolean
  Memory : Memory  InheritSampleTime=on  LinearizeAsDelay=on
  Sum1 : Sum  Inputs=+-+
  XOR{,1..3} (4 alike) : Logic  Operator=XOR  IconShape=distinctive  AllPortsSameDT=off  OutDataTypeStr=boolean
  Signal Delayed : Outport
  wires:
  Sum1/1 -> Memory/1, Signal Delayed/1
  Data Type Conversion1/1 -> Sum1/2
  Memory/1 -> Sum1/3
  Signal/1 -> Detect Fall Nonpositive/1, Detect Rise Positive/1
  Data Type Conversion2/1 -> Sum1/1
  Detect Fall Nonpositive/1 -> Delay1/1
  Detect Rise Positive/1 -> Delay/1
  Delay1/1 -> XOR/2, AND/2
  Delay/1 -> XOR1/1, AND/1
  XOR1/1 -> Delay2/1
  AND/1 -> XOR1/2, XOR/1
  Delay2/1 -> XOR3/1, AND1/1
  AND1/1 -> XOR3/2, XOR2/1
  XOR/1 -> XOR2/2, AND1/2
  XOR3/1 -> Data Type Conversion2/1
  XOR2/1 -> Data Type Conversion1/1

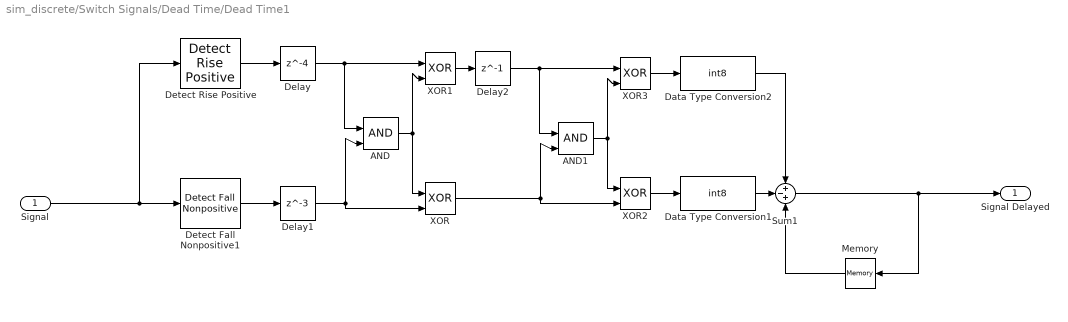
== system sim_discrete/Switch Signals/Dead Time/Dead Time1 ==
  Signal : Inport
  AND : Logic  IconShape=distinctive  AllPortsSameDT=off  OutDataTypeStr=boolean
  AND1 : Logic  IconShape=distinctive  AllPortsSameDT=off  OutDataTypeStr=boolean
  Data Type Conversion1 : DataTypeConversion  OutDataTypeStr=int8
  Data Type Conversion2 : DataTypeConversion  OutDataTypeStr=int8
  Delay : Delay  DelayLength=4
  Delay1 : Delay  DelayLength=3
  Delay2 : Delay  DelayLength=1
  Detect Fall Nonpositive1 : simulink/Logic and Bit Operations/Detect Fall Nonpositive  vinit=true  OutDataTypeStr=boolean
      settings: SourceProductName=Simulink  SourceProductBaseCode=SL
  Detect Rise Positive : simulink/Logic and Bit Operations/Detect Rise Positive  vinit=0  OutDataTypeStr=boolean
  Memory : Memory  InheritSampleTime=on  LinearizeAsDelay=on
  Sum1 : Sum  Inputs=+-+
  XOR{,1..3} (4 alike) : Logic  Operator=XOR  IconShape=distinctive  AllPortsSameDT=off  OutDataTypeStr=boolean
  Signal Delayed : Outport
  wires:
  Sum1/1 -> Memory/1, Signal Delayed/1
  Data Type Conversion1/1 -> Sum1/2
  Memory/1 -> Sum1/3
  Signal/1 -> Detect Fall Nonpositive1/1, Detect Rise Positive/1
  Data Type Conversion2/1 -> Sum1/1
  Detect Fall Nonpositive1/1 -> Delay1/1
  Detect Rise Positive/1 -> Delay/1
  Delay1/1 -> XOR/2, AND/2
  Delay/1 -> XOR1/1, AND/1
  XOR1/1 -> Delay2/1
  AND/1 -> XOR1/2, XOR/1
  Delay2/1 -> XOR3/1, AND1/1
  AND1/1 -> XOR3/2, XOR2/1
  XOR/1 -> XOR2/2, AND1/2
  XOR3/1 -> Data Type Conversion2/1
  XOR2/1 -> Data Type Conversion1/1

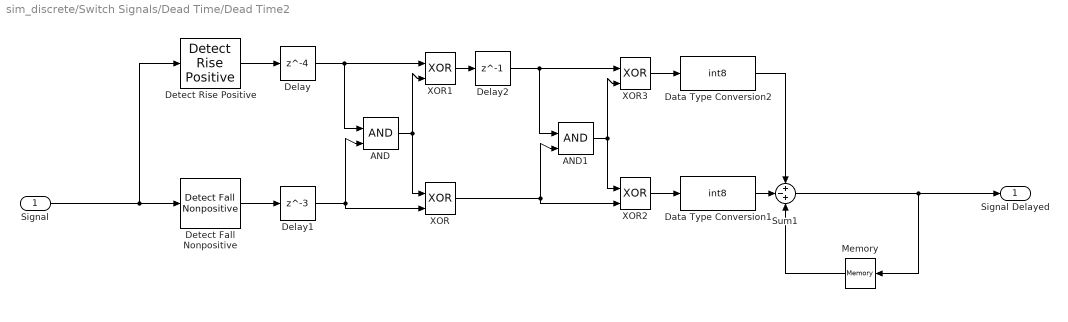
== system sim_discrete/Switch Signals/Dead Time/Dead Time2 ==
  Signal : Inport
  AND : Logic  IconShape=distinctive  AllPortsSameDT=off  OutDataTypeStr=boolean
  AND1 : Logic  IconShape=distinctive  AllPortsSameDT=off  OutDataTypeStr=boolean
  Data Type Conversion1 : DataTypeConversion  OutDataTypeStr=int8
  Data Type Conversion2 : DataTypeConversion  OutDataTypeStr=int8
  Delay : Delay  DelayLength=4
  Delay1 : Delay  DelayLength=3
  Delay2 : Delay  DelayLength=1
  Detect Fall Nonpositive : simulink/Logic and Bit Operations/Detect Fall Nonpositive  vinit=true  OutDataTypeStr=boolean
      settings: SourceProductName=Simulink  SourceProductBaseCode=SL
  Detect Rise Positive : simulink/Logic and Bit Operations/Detect Rise Positive  vinit=0  OutDataTypeStr=boolean
  Memory : Memory  InheritSampleTime=on  LinearizeAsDelay=on
  Sum1 : Sum  Inputs=+-+
  XOR{,1..3} (4 alike) : Logic  Operator=XOR  IconShape=distinctive  AllPortsSameDT=off  OutDataTypeStr=boolean
  Signal Delayed : Outport
  wires:
  Sum1/1 -> Memory/1, Signal Delayed/1
  Data Type Conversion1/1 -> Sum1/2
  Memory/1 -> Sum1/3
  Signal/1 -> Detect Fall Nonpositive/1, Detect Rise Positive/1
  Data Type Conversion2/1 -> Sum1/1
  Detect Fall Nonpositive/1 -> Delay1/1
  Detect Rise Positive/1 -> Delay/1
  Delay1/1 -> XOR/2, AND/2
  Delay/1 -> XOR1/1, AND/1
  XOR1/1 -> Delay2/1
  AND/1 -> XOR1/2, XOR/1
  Delay2/1 -> XOR3/1, AND1/1
  AND1/1 -> XOR3/2, XOR2/1
  XOR/1 -> XOR2/2, AND1/2
  XOR3/1 -> Data Type Conversion2/1
  XOR2/1 -> Data Type Conversion1/1

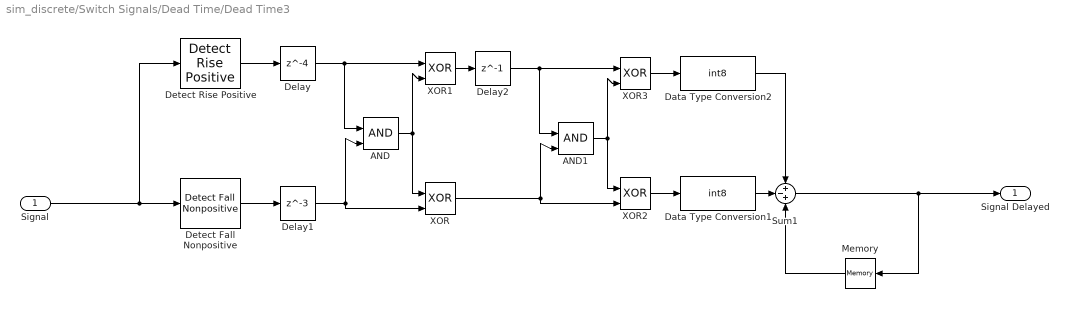
== system sim_discrete/Switch Signals/Dead Time/Dead Time3 ==
  Signal : Inport
  AND : Logic  IconShape=distinctive  AllPortsSameDT=off  OutDataTypeStr=boolean
  AND1 : Logic  IconShape=distinctive  AllPortsSameDT=off  OutDataTypeStr=boolean
  Data Type Conversion1 : DataTypeConversion  OutDataTypeStr=int8
  Data Type Conversion2 : DataTypeConversion  OutDataTypeStr=int8
  Delay : Delay  DelayLength=4
  Delay1 : Delay  DelayLength=3
  Delay2 : Delay  DelayLength=1
  Detect Fall Nonpositive : simulink/Logic and Bit Operations/Detect Fall Nonpositive  vinit=true  OutDataTypeStr=boolean
      settings: SourceProductName=Simulink  SourceProductBaseCode=SL
  Detect Rise Positive : simulink/Logic and Bit Operations/Detect Rise Positive  vinit=0  OutDataTypeStr=boolean
  Memory : Memory  InheritSampleTime=on  LinearizeAsDelay=on
  Sum1 : Sum  Inputs=+-+
  XOR{,1..3} (4 alike) : Logic  Operator=XOR  IconShape=distinctive  AllPortsSameDT=off  OutDataTypeStr=boolean
  Signal Delayed : Outport
  wires:
  Sum1/1 -> Memory/1, Signal Delayed/1
  Data Type Conversion1/1 -> Sum1/2
  Memory/1 -> Sum1/3
  Signal/1 -> Detect Rise Positive/1, Detect Fall Nonpositive/1
  Data Type Conversion2/1 -> Sum1/1
  Detect Fall Nonpositive/1 -> Delay1/1
  Detect Rise Positive/1 -> Delay/1
  Delay1/1 -> XOR/2, AND/2
  Delay/1 -> XOR1/1, AND/1
  XOR1/1 -> Delay2/1
  AND/1 -> XOR1/2, XOR/1
  Delay2/1 -> XOR3/1, AND1/1
  AND1/1 -> XOR3/2, XOR2/1
  XOR/1 -> XOR2/2, AND1/2
  XOR3/1 -> Data Type Conversion2/1
  XOR2/1 -> Data Type Conversion1/1

== system sim_discrete/Reference Manager/Reference Update/Equilibrium Current Determination/Current Correction ==
  IL_e : Inport
  Vref : Inport  Port=2
  Vo : Inport  Port=3
  Constant : Constant  Value=0
  Current Correction Step : Step  Time=current_correction_start  SampleTime=0
  PID Controller : simulink/Continuous/PID Controller  Controller=I  TimeDomain=Continuous-time  SampleTime=-1  IntegratorMethod=Forward Euler  FilterMethod=Forward Euler  Form=Parallel  UseFilter=on  ControllerParametersSource=internal  P=0  I=5  D=0  N=100  InitialConditionSource=internal  InitialConditionForIntegrator=0  InitialConditionForFilter=0  ExternalReset=none  LimitOutput=off  UpperSaturationLimit=inf  LowerSaturationLimit=-inf  LinearizeAsGain=on  AntiWindupMode=none  Kb=1  TrackingMode=off  Kt=1  PParamMin=[]  PParamMax=[]  IParamMin=[]  IParamMax=[]  DParamMin=[]  DParamMax=[]  NParamMin=[]  NParamMax=[]  KbParamMin=[]  KbParamMax=[]  KtParamMin=[]  KtParamMax=[]  POutMin=[]  POutMax=[]  IOutMin=[]  IOutMax=[]  DOutMin=[]  DOutMax=[]  NOutMin=[]  NOutMax=[]  KbOutMin=[]  KbOutMax=[]  KtOutMin=[]  KtOutMax=[]  IntegratorOutMin=[]  IntegratorOutMax=[]  FilterOutMin=[]  FilterOutMax=[]  SumOutMin=[]  SumOutMax=[]  SumI1OutMin=[]  SumI1OutMax=[]  SumI2OutMin=[]  SumI2OutMax=[]  SumI3OutMin=[]  SumI3OutMax=[]  SumDOutMin=[]  SumDOutMax=[]  SaturationOutMin=[]  SaturationOutMax=[]  IntegratorContinuousStateAttributes=''  IntegratorStateMustResolveToSignalObject=off  IntegratorRTWStateStorageClass=Auto  FilterContinuousStateAttributes=''  FilterStateMustResolveToSignalObject=off  FilterRTWStateStorageClass=Auto  DifferentiatorICPrevScaledInput=0  DifferentiatorOutMin=[]  DifferentiatorOutMax=[]  FilterDiffOutCoefMin=[]  FilterDiffOutCoefMax=[]  SumDenOutMin=[]  SumDenOutMax=[]  SumNumOutMin=[]  SumNumOutMax=[]  ReciprocalOutMin=[]  ReciprocalOutMax=[]  DivideOutMin=[]  DivideOutMax=[]  TunerSelectOption=Transfer Function Based (PID Tuner App)
  Sum : Sum  Inputs=++|
  Sum1 : Sum  Inputs=-+|
  Switch : Switch  Criteria=u2 > Threshold
  Ie : Outport
  wires:
  Vo/1 -> Sum1/1
  PID Controller/1 -> Sum/2
  Sum/1 -> Ie/1
  Vref/1 -> Sum1/2
  IL_e/1 -> Sum/1
  Switch/1 -> PID Controller/1
  Current Correction Step/1 -> Switch/2
  Sum1/1 -> Switch/1
  Constant/1 -> Switch/3

== system sim_discrete/Reference Manager/Reference Update/Equilibrium Current Determination/Current Estimation ==
  Ve : Inport
  Vin : Inport  Port=2
  Boost : Subsystem
  Buck : Subsystem
  Buck-Boost : Subsystem
  Buck-Boost 3 : Subsystem
  Multiport Switch : MultiPortSwitch  Inputs=4
  Ie : Outport
  wires:
  Multiport Switch/1 -> Ie/1
  [converter_index] -> Multiport Switch/1
  Buck-Boost 3/1(Ie) -> Multiport Switch/5
  Boost/1(Ie) -> Multiport Switch/3
  Buck-Boost/1(Ie) -> Multiport Switch/4
  Buck/1(Ie) -> Multiport Switch/2
  Ve/1 -> Boost/2(Vin), Buck/1(Ve), Buck-Boost 3/1(Ve), Buck-Boost/1(Ve)
  Vin/1 -> Boost/1(Ve), Buck/2(Vin), Buck-Boost 3/2(Vin), Buck-Boost/2(Vin)

== system sim_discrete/Reference Manager/Reference Update/Equilibrium Current Determination/Current Estimation/Boost ==
  Ve : Inport
  Vin : Inport  Port=2
  Boost Equilibrium Current : MATLAB Function  TreatAsAtomicUnit=on
  Constant : Constant  Value=R
  Constant1 : Constant  Value=Ro
  Ie : Outport
  wires:
  Constant1/1 -> Boost Equilibrium Current/4(Ro)
  Constant/1 -> Boost Equilibrium Current/3(R)
  Vin/1 -> Boost Equilibrium Current/2(Vin)
  Boost Equilibrium Current/1(I) -> Ie/1
  Ve/1 -> Boost Equilibrium Current/1(Ve)

== system sim_discrete/Reference Manager/Reference Update/Equilibrium Current Determination/Current Estimation/Buck ==
  Ve : Inport
  Vin : Inport  Port=2
  Buck Equilibrium Current : MATLAB Function  TreatAsAtomicUnit=on
  Constant : Constant  Value=R
  Constant1 : Constant  Value=Ro
  Ie : Outport
  wires:
  Constant1/1 -> Buck Equilibrium Current/4(Ro)
  Constant/1 -> Buck Equilibrium Current/3(R)
  Vin/1 -> Buck Equilibrium Current/2(Vin)
  Buck Equilibrium Current/1(I) -> Ie/1
  Ve/1 -> Buck Equilibrium Current/1(Ve)

== system sim_discrete/Reference Manager/Reference Update/Equilibrium Current Determination/Current Estimation/Buck-Boost ==
  Ve : Inport
  Vin : Inport  Port=2
  Buck-Boost Equilibrium Current : MATLAB Function  TreatAsAtomicUnit=on
  Constant : Constant  Value=R
  Constant1 : Constant  Value=Ro
  Ie : Outport
  wires:
  Constant1/1 -> Buck-Boost Equilibrium Current/4(Ro)
  Constant/1 -> Buck-Boost Equilibrium Current/3(R)
  Vin/1 -> Buck-Boost Equilibrium Current/2(Vin)
  Buck-Boost Equilibrium Current/1(I) -> Ie/1
  Ve/1 -> Buck-Boost Equilibrium Current/1(Ve)

== system sim_discrete/Reference Manager/Reference Update/Equilibrium Current Determination/Current Estimation/Buck-Boost 3 ==
  Ve : Inport
  Vin : Inport  Port=2
  Buck-Boost Equilibrium Current : MATLAB Function  TreatAsAtomicUnit=on
  Constant : Constant  Value=R
  Constant1 : Constant  Value=Ro
  Ie : Outport
  wires:
  Constant1/1 -> Buck-Boost Equilibrium Current/4(Ro)
  Constant/1 -> Buck-Boost Equilibrium Current/3(R)
  Vin/1 -> Buck-Boost Equilibrium Current/2(Vin)
  Buck-Boost Equilibrium Current/1(I) -> Ie/1
  Ve/1 -> Buck-Boost Equilibrium Current/1(Ve)

== matlab function sim_discrete/Reference Manager/Reference Update/Equilibrium Current Determination/Current Estimation/Boost/Boost Equilibrium Current ==
  data: Ve input; I output; Vin input; R input; Ro input
function I = EquilibriumCurrent(Ve, Vin, R, Ro)
    I = Vin/(2*R) - sqrt( Vin^2/(4*R^2) - Ve^2/(R*Ro) );
end

== matlab function sim_discrete/Reference Manager/Reference Update/Equilibrium Current Determination/Current Estimation/Buck-Boost 3/Buck-Boost Equilibrium Current ==
  data: Ve input; I output; Vin input; R input; Ro input
function I = EquilibriumCurrent(Ve, Vin, R, Ro)
    I = Vin/(2*R) - sqrt( Vin^2/(4*R^2) - Ve*(Ve+Vin)/(R*Ro) );
end

== matlab function sim_discrete/Reference Manager/Reference Update/Equilibrium Current Determination/Current Estimation/Buck/Buck Equilibrium Current ==
  data: Ve input; I output; Vin input; R input; Ro input
function I = EquilibriumCurrent(Ve, Vin, R, Ro)
    I = Ve/Ro;
end

== matlab function sim_discrete/Reference Manager/Reference Update/Equilibrium Current Determination/Current Estimation/Buck-Boost/Buck-Boost Equilibrium Current ==
  data: Ve input; I output; Vin input; R input; Ro input
function I = EquilibriumCurrent(Ve, Vin, R, Ro)
    I = Vin/(2*R) - sqrt( Vin^2/(4*R^2) - Ve*(Ve+Vin)/(R*Ro) );
end

== matlab function sim_discrete/Controller/Discrete Switched Control/Discrete Switching Strategy ==
  data: theorem input; sys input; x input; u input; k output; xe input
function k = discrete_switching_strategy(theorem, sys, x, u, xe)
    Xi = x - xe;
    sig = zeros(sys.N,1);
    
    d = sys.h'/sys.P*sys.h;
    for i=1:sys.N
        switch(theorem)
            case 1
                Xipp = sys.A(:,:,i)*Xi + sys.L(:,:,i)*u;
                sig(i) = [1 Xipp'] * [d sys.h'; sys.h sys.P] * [1; Xipp];
            case 2
                Xipp = sys.A(:,:,i)*Xi + sys.L(:,:,i)*u;
                sig(i) = [1 Xipp'] * [d sys.h'; sys.h sys.P] * [1; Xipp];
        end
    end
    [~, k] = min(sig);
end
